simulink model "dm_1_and_2points"  (R2018a)
settings: Solver=VariableStepAuto  StartTime=0.0  StopTime=tf  RelTol=1e-3
values from neighbouring files (symbols this model uses):
  A = -m*(lf*Kf-lr*Kr)/2/l/l/Kr/Kf    (= 0.00110674647712)    [driver_model.m]
  dt = 0.001    [driver_model.m]
  G1 = 2*omega*omega*(1-2*xi*xi)/V/(Tp1*Tp1*omega*omega-4*omega*xi*Tp1+2)    (= -0.886921257181)    [driver_model.m]
  G2 = omega*omega*(omega*Tp1-2*xi)^2/V/(Tp1*Tp1*omega*omega-4*omega*xi*Tp1+2)    (= 5.08596125718)    [driver_model.m]
  h = (1+A*V*V)*l/V    (= 0.180205985784)    [driver_model.m]
  h1 = 2*V/lp/lp    (= 0.288)    [driver_model.m]
  I = 2500    [driver_model.m]
  Kf = 55000    [driver_model.m]
  Kr = 60000    [driver_model.m]
  l = lf+lr    (= 2.7)    [driver_model.m]
  lf = 1.1    [driver_model.m]
  lp = tp*V    (= 13.8888888889)    [driver_model.m]
  lp1 = Tp1*V    (= 33.3333333333)    [driver_model.m]
  lp2 = Tp2*V    (= 14.3068415638)    [driver_model.m]
  lr = 1.6    [driver_model.m]
  m = 1500    [driver_model.m]
  n = 18.7    [driver_model.m]
  tau = 0.0    (= 0)    [driver_model.m]
  V = 100/3.6    (= 27.7777777778)    [driver_model.m]
  y0 = 2.0    (= 2)    [driver_model.m]
libraries: simulink x5
settings Model: Creator=aoki-soya  LastModifiedBy=aoki-soya

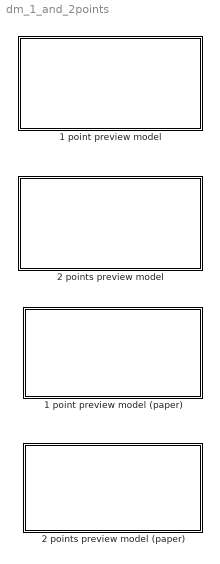
== system dm_1_and_2points ==
  1 point preview model : Subsystem
  1 point preview model (paper) : Subsystem
  2 points preview model : Subsystem
  2 points preview model (paper) : Subsystem

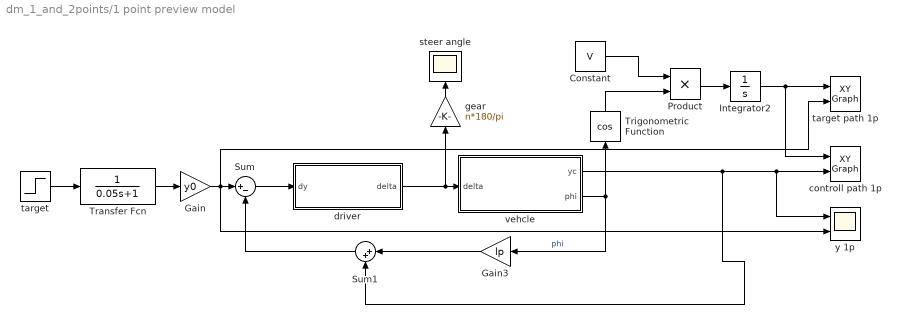
== system dm_1_and_2points/1 point preview model ==
  Constant : Constant  Value=V
  Gain : Gain  Gain=y0
  Gain3 : Gain  Gain=lp
  Integrator2 : Integrator
  Product : Product
  Sum : Sum  Inputs=|+-
  Sum1 : Sum  Inputs=|++
  Transfer Fcn : TransferFcn  Denominator=[0.05 1]
  Trigonometric Function : Trigonometry  Operator=cos
  controll path 1p : simulink/Sinks/XY Graph  xmin=-1  xmax=V*tf+10  ymin=-1  ymax=y0*2  st=-1
  driver : Subsystem
  gear : Gain  Gain=n*180/pi
  steer angle : Scope
  "target " : Step  SampleTime=dt
  target path 1p : simulink/Sinks/XY Graph  xmin=-1  xmax=V*tf+10  ymin=-1  ymax=y0*2  st=-1
  vehcle : Subsystem
  y 1p : Scope  NumInputPorts=2
  wires:
  Sum1/1 -> Sum/2
  Product/1 -> Integrator2/1
  vehcle/1(yc) -> Sum1/2, y 1p/1, controll path 1p/2
  gear/1 -> steer angle/1
  Gain/1 -> target path 1p/2, y 1p/2, Sum/1
  "target "/1 -> Transfer Fcn/1
  vehcle/2(phi) -> Gain3/1, Trigonometric Function/1  "phi"
  Constant/1 -> Product/1
  Trigonometric Function/1 -> Product/2
  Integrator2/1 -> controll path 1p/1, target path 1p/1
  Gain3/1 -> Sum1/1
  Transfer Fcn/1 -> Gain/1
  driver/1(delta) -> gear/1, vehcle/1(delta)
  Sum/1 -> driver/1(dy)

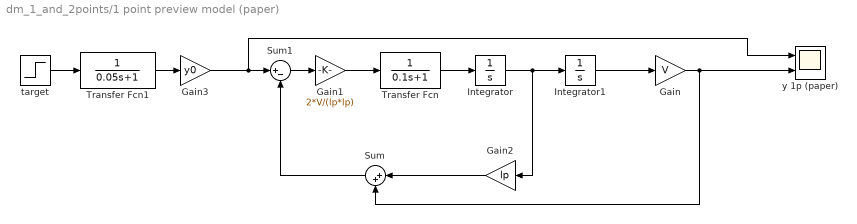
== system dm_1_and_2points/1 point preview model (paper) ==
  Gain : Gain  Gain=V
  Gain1 : Gain  Gain=2*V/(lp*lp)
  Gain2 : Gain  Gain=lp
  Gain3 : Gain  Gain=y0
  Integrator : Integrator
  Integrator1 : Integrator
  Sum : Sum  Inputs=|++
  Sum1 : Sum  Inputs=|+-
  Transfer Fcn : TransferFcn  Denominator=[0.1 1]
  Transfer Fcn1 : TransferFcn  Denominator=[0.05 1]
  "target " : Step  SampleTime=dt
  y 1p (paper) : Scope  NumInputPorts=2
  wires:
  Gain1/1 -> Transfer Fcn/1
  Transfer Fcn/1 -> Integrator/1
  Integrator1/1 -> Gain/1
  Integrator/1 -> Gain2/1, Integrator1/1
  Gain2/1 -> Sum/1
  Gain/1 -> y 1p (paper)/2, Sum/2
  Gain3/1 -> y 1p (paper)/1, Sum1/1
  Sum1/1 -> Gain1/1
  Sum/1 -> Sum1/2
  Transfer Fcn1/1 -> Gain3/1
  "target "/1 -> Transfer Fcn1/1

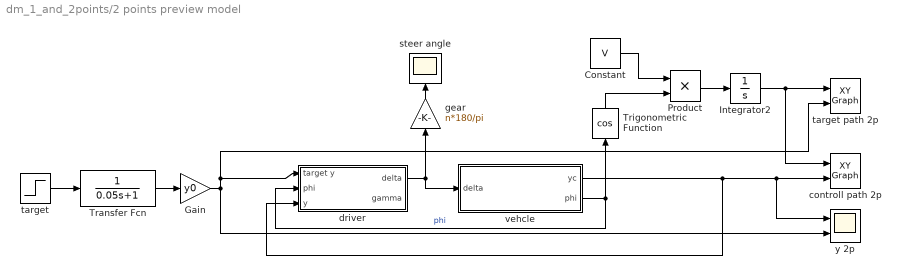
== system dm_1_and_2points/2 points preview model ==
  Constant : Constant  Value=V
  Gain : Gain  Gain=y0
  Integrator2 : Integrator
  Product : Product
  Transfer Fcn : TransferFcn  Denominator=[0.05 1]
  Trigonometric Function : Trigonometry  Operator=cos
  controll path 2p : simulink/Sinks/XY Graph  xmin=-1  xmax=V*tf+10  ymin=-1  ymax=y0*2  st=-1
  driver : Subsystem
  gear : Gain  Gain=n*180/pi
  steer angle : Scope
  "target " : Step  SampleTime=dt
  target path 2p : simulink/Sinks/XY Graph  xmin=-1  xmax=V*tf+10  ymin=-1  ymax=y0*2  st=-1
  vehcle : Subsystem
  y 2p : Scope  NumInputPorts=2
  wires:
  Product/1 -> Integrator2/1
  vehcle/1(yc) -> driver/3(y), y 2p/1, controll path 2p/2
  gear/1 -> steer angle/1
  "target "/1 -> Transfer Fcn/1
  vehcle/2(phi) -> driver/2(phi), Trigonometric Function/1  "phi"
  Constant/1 -> Product/1
  Trigonometric Function/1 -> Product/2
  Integrator2/1 -> controll path 2p/1, target path 2p/1
  Transfer Fcn/1 -> Gain/1
  driver/1(delta) -> vehcle/1(delta), gear/1
  Gain/1 -> driver/1(target y), target path 2p/2, y 2p/2

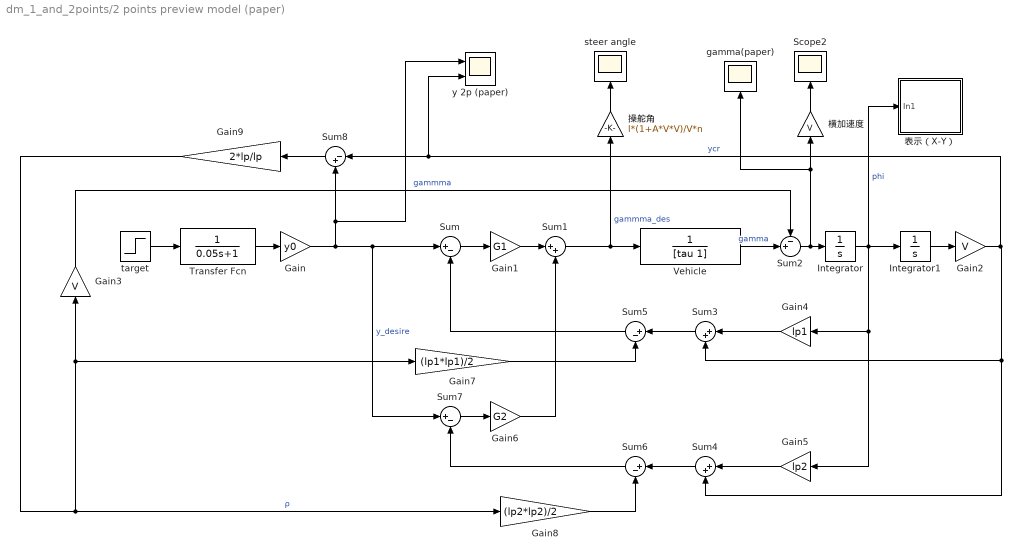
== system dm_1_and_2points/2 points preview model (paper) ==
  Gain : Gain  Gain=y0
  Gain1 : Gain  Gain=G1
  Gain2 : Gain  Gain=V
  Gain3 : Gain  Gain=V
  Gain4 : Gain  Gain=lp1
  Gain5 : Gain  Gain=lp2
  Gain6 : Gain  Gain=G2
  Gain7 : Gain  Gain=(lp1*lp1)/2
  Gain8 : Gain  Gain=(lp2*lp2)/2
  Gain9 : Gain  Gain=2*lp/lp
  Integrator : Integrator
  Integrator1 : Integrator
  Scope2 : Scope
  Sum{,5..7} (4 alike) : Sum  Inputs=|+-
  Sum1 : Sum  Inputs=|++
  Sum2 : Sum  Inputs=-+|
  Sum3 : Sum  Inputs=|++
  Sum4 : Sum  Inputs=|++
  Sum8 : Sum  Inputs=|-+
  Transfer Fcn : TransferFcn  Denominator=[0.05 1]
  Vehicle : TransferFcn  Denominator=[tau 1]
  gamma(paper) : Scope
  steer angle : Scope
  "target " : Step  SampleTime=dt
  y 2p (paper) : Scope  NumInputPorts=2
  操舵角 : Gain  Gain=l*(1+A*V*V)/V*n
  横加速度 : Gain  Gain=V
  表示（X-Y） : Subsystem
  wires:
  Gain7/1 -> Sum5/2
  Sum/1 -> Gain1/1
  Sum3/1 -> Sum5/1
  Sum5/1 -> Sum/2
  Gain4/1 -> Sum3/1
  Gain1/1 -> Sum1/1
  Gain6/1 -> Sum1/2
  Gain8/1 -> Sum6/2
  Sum4/1 -> Sum6/1
  Gain5/1 -> Sum4/1
  Vehicle/1 -> Sum2/2  "gamma"
  Integrator1/1 -> Gain2/1
  Integrator/1 -> 表示（X-Y）/1(In1), Gain5/1, Gain4/1, Integrator1/1  "phi"
  Sum6/1 -> Sum7/2
  Sum7/1 -> Gain6/1
  Gain3/1 -> Sum2/1  "gammma"
  Sum1/1 -> Vehicle/1, 操舵角/1  "gammma_des"
  Gain2/1 -> y 2p (paper)/2, Sum8/1, Sum4/2, Sum3/2  "ycr"
  Gain9/1 -> Gain8/1, Gain3/1, Gain7/1  "ρ"
  Gain/1 -> y 2p (paper)/1, Sum8/2, Sum/1, Sum7/1  "y_desire"
  Sum8/1 -> Gain9/1
  操舵角/1 -> steer angle/1
  Sum2/1 -> gamma(paper)/1, 横加速度/1, Integrator/1
  横加速度/1 -> Scope2/1
  Transfer Fcn/1 -> Gain/1
  "target "/1 -> Transfer Fcn/1

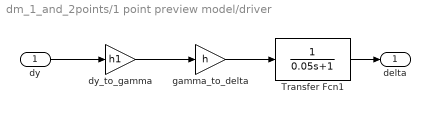
== system dm_1_and_2points/1 point preview model/driver ==
  dy : Inport
  Transfer Fcn1 : TransferFcn  Denominator=[0.05 1]
  dy_to_gamma : Gain  Gain=h1
  gamma_to_delta : Gain  Gain=h
  delta : Outport
  wires:
  Transfer Fcn1/1 -> delta/1
  dy/1 -> dy_to_gamma/1
  gamma_to_delta/1 -> Transfer Fcn1/1
  dy_to_gamma/1 -> gamma_to_delta/1

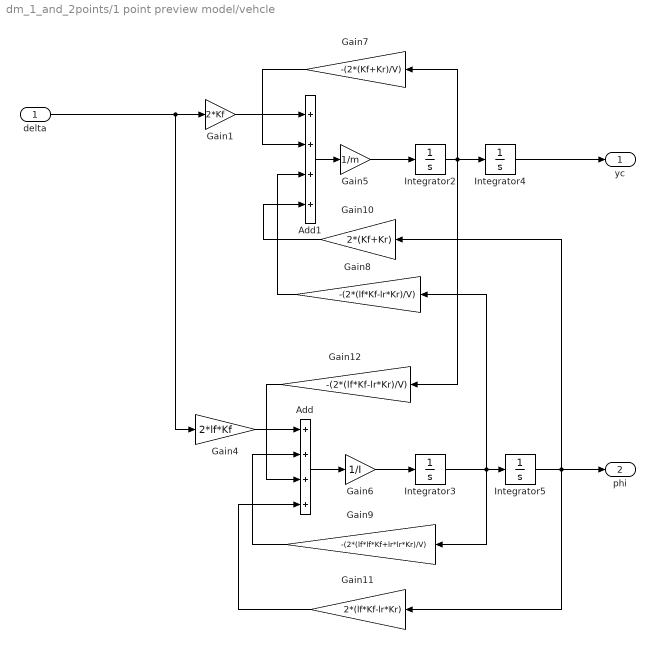
== system dm_1_and_2points/1 point preview model/vehcle ==
  delta : Inport
  Add : Sum  Inputs=++++
  Add1 : Sum  Inputs=++++
  Gain1 : Gain  Gain=2*Kf
  Gain10 : Gain  Gain=2*(Kf+Kr)
  Gain11 : Gain  Gain=2*(lf*Kf-lr*Kr)
  Gain12 : Gain  Gain=-(2*(lf*Kf-lr*Kr)/V)
  Gain4 : Gain  Gain=2*lf*Kf
  Gain5 : Gain  Gain=1/m
  Gain6 : Gain  Gain=1/I
  Gain7 : Gain  Gain=-(2*(Kf+Kr)/V)
  Gain8 : Gain  Gain=-(2*(lf*Kf-lr*Kr)/V)
  Gain9 : Gain  Gain=-(2*(lf*lf*Kf+lr*lr*Kr)/V)
  Integrator{2..5} (4 alike) : Integrator
  yc : Outport
  phi : Outport  Port=2
  wires:
  Gain6/1 -> Integrator3/1
  Integrator4/1 -> yc/1
  Add/1 -> Gain6/1
  Gain10/1 -> Add1/4
  Add1/1 -> Gain5/1
  Gain11/1 -> Add/4
  Gain8/1 -> Add1/3
  Gain5/1 -> Integrator2/1
  Gain1/1 -> Add1/1
  Gain9/1 -> Add/2
  Integrator3/1 -> Gain8/1, Integrator5/1, Gain9/1
  Integrator2/1 -> Gain7/1, Gain12/1, Integrator4/1
  Gain4/1 -> Add/1
  Gain12/1 -> Add/3
  Integrator5/1 -> phi/1, Gain11/1, Gain10/1
  Gain7/1 -> Add1/2
  delta/1 -> Gain4/1, Gain1/1

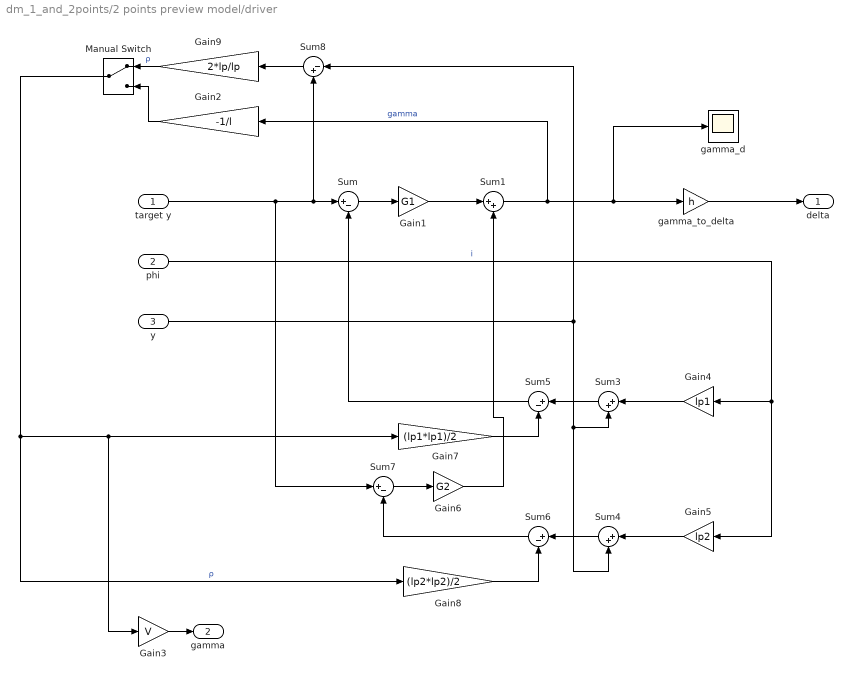
== system dm_1_and_2points/2 points preview model/driver ==
  target y : Inport
  phi : Inport  Port=2
  y : Inport  Port=3
  Gain1 : Gain  Gain=G1
  Gain2 : Gain  Gain=-1/l
  Gain3 : Gain  Gain=V
  Gain4 : Gain  Gain=lp1
  Gain5 : Gain  Gain=lp2
  Gain6 : Gain  Gain=G2
  Gain7 : Gain  Gain=(lp1*lp1)/2
  Gain8 : Gain  Gain=(lp2*lp2)/2
  Gain9 : Gain  Gain=2*lp/lp
  Manual Switch : ManualSwitch
  Sum{,5..7} (4 alike) : Sum  Inputs=|+-
  Sum1 : Sum  Inputs=|++
  Sum3 : Sum  Inputs=|++
  Sum4 : Sum  Inputs=|++
  Sum8 : Sum  Inputs=|-+
  gamma_d : Scope
  gamma_to_delta : Gain  Gain=h
  delta : Outport
  gamma : Outport  Port=2
  wires:
  Sum7/1 -> Gain6/1
  Sum3/1 -> Sum5/1
  Sum4/1 -> Sum6/1
  Sum5/1 -> Sum/2
  y/1 -> Sum8/1, Sum4/2, Sum3/2
  Gain4/1 -> Sum3/1
  Gain6/1 -> Sum1/2
  target y/1 -> Sum7/1, Sum8/2, Sum/1
  Gain7/1 -> Sum5/2
  Gain8/1 -> Sum6/2
  Gain5/1 -> Sum4/1
  phi/1 -> Gain5/1, Gain4/1  "i"
  Manual Switch/1 -> Gain8/1, Gain3/1, Gain7/1  "ρ"
  Sum6/1 -> Sum7/2
  Sum8/1 -> Gain9/1
  Gain1/1 -> Sum1/1
  Sum/1 -> Gain1/1
  Sum1/1 -> Gain2/1, gamma_d/1, gamma_to_delta/1  "gamma"
  gamma_to_delta/1 -> delta/1
  Gain3/1 -> gamma/1
  Gain9/1 -> Manual Switch/1  "ρ"
  Gain2/1 -> Manual Switch/2

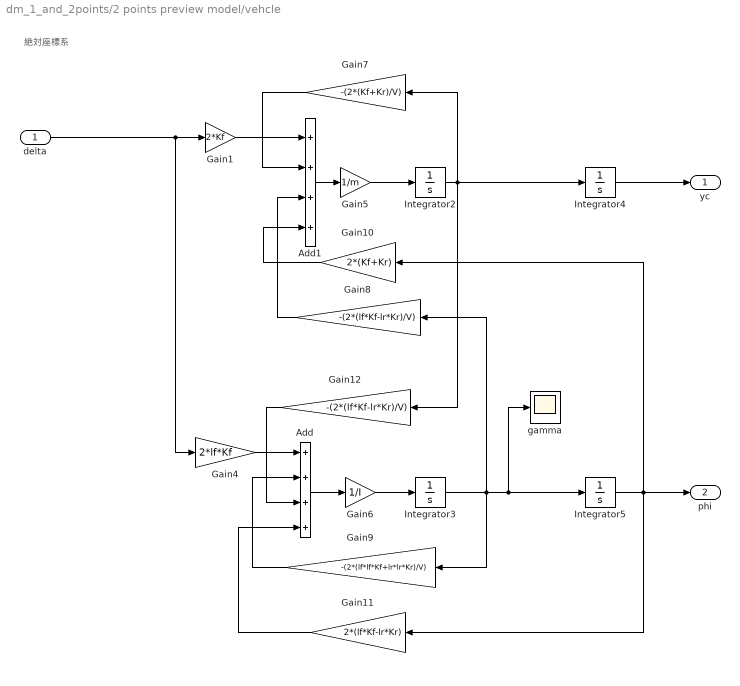
== system dm_1_and_2points/2 points preview model/vehcle ==
  note: 絶対座標系
  delta : Inport
  Add : Sum  Inputs=++++
  Add1 : Sum  Inputs=++++
  Gain1 : Gain  Gain=2*Kf
  Gain10 : Gain  Gain=2*(Kf+Kr)
  Gain11 : Gain  Gain=2*(lf*Kf-lr*Kr)
  Gain12 : Gain  Gain=-(2*(lf*Kf-lr*Kr)/V)
  Gain4 : Gain  Gain=2*lf*Kf
  Gain5 : Gain  Gain=1/m
  Gain6 : Gain  Gain=1/I
  Gain7 : Gain  Gain=-(2*(Kf+Kr)/V)
  Gain8 : Gain  Gain=-(2*(lf*Kf-lr*Kr)/V)
  Gain9 : Gain  Gain=-(2*(lf*lf*Kf+lr*lr*Kr)/V)
  Integrator{2..5} (4 alike) : Integrator
  gamma : Scope
  yc : Outport
  phi : Outport  Port=2
  wires:
  Gain6/1 -> Integrator3/1
  Integrator4/1 -> yc/1
  Add/1 -> Gain6/1
  Gain10/1 -> Add1/4
  Add1/1 -> Gain5/1
  Gain11/1 -> Add/4
  Gain8/1 -> Add1/3
  Gain5/1 -> Integrator2/1
  Gain1/1 -> Add1/1
  Gain9/1 -> Add/2
  Integrator2/1 -> Gain7/1, Gain12/1, Integrator4/1
  Gain4/1 -> Add/1
  Gain12/1 -> Add/3
  Integrator5/1 -> phi/1, Gain11/1, Gain10/1
  Gain7/1 -> Add1/2
  delta/1 -> Gain4/1, Gain1/1
  Integrator3/1 -> Integrator5/1, gamma/1, Gain8/1, Gain9/1

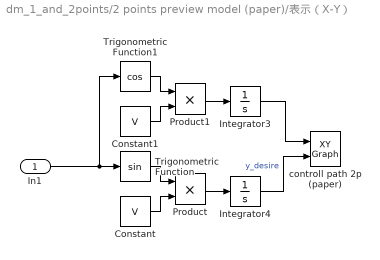
== system dm_1_and_2points/2 points preview model (paper)/表示（X-Y） ==
  In1 : Inport
  Constant : Constant  Value=V
  Constant1 : Constant  Value=V
  Integrator3 : Integrator
  Integrator4 : Integrator
  Product : Product
  Product1 : Product
  Trigonometric Function : Trigonometry
  Trigonometric Function1 : Trigonometry  Operator=cos
  controll path 2p (paper) : simulink/Sinks/XY Graph  xmin=-1  xmax=V*tf  ymin=-1  ymax=y0*2  st=-1
  wires:
  Integrator4/1 -> controll path 2p (paper)/2  "y_desire"
  Product/1 -> Integrator4/1
  Constant1/1 -> Product1/2
  Product1/1 -> Integrator3/1
  Trigonometric Function/1 -> Product/1
  Trigonometric Function1/1 -> Product1/1
  Integrator3/1 -> controll path 2p (paper)/1
  In1/1 -> Trigonometric Function1/1, Trigonometric Function/1
  Constant/1 -> Product/2
